simulink model "practice_final_part_5"  (Simulink 8.3)
settings: Solver=ode45  StartTime=0.0  StopTime=20  RelTol=1e-3
undefined symbols (not defined in the file or in its folder): ctrl_est, drawRodMass, P
settings Model: Creator=beard  LastModifiedBy=jhl48
settings DataIOCC: LimitDataPoints=off
settings OptimizationCC: ExpressionDepthLimit=2147483647
settings DebuggingCC: SolverPrmCheckMsg=none  FcnCallInpInsideContextMsg=UseLocalSettings

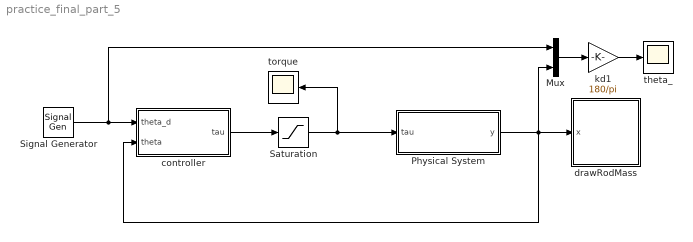
== system practice_final_part_5 ==
  Mux : Mux  Inputs=2
  Physical System : Subsystem
  Saturation : Saturate  UpperLimit=P.tau_max  LowerLimit=-P.tau_max
  Signal Generator : SignalGenerator  WaveForm=square  Amplitude=10*pi/180  Frequency=.1
  controller : Subsystem
  drawRodMass : Subsystem
      mask init:
      | % drawing parameters
      | L = 1;
      | w = 0.01;
      | R = 0.1;
      | H = 1;
      mask Display: image(imread('tv.jpg'))
  kd1 : Gain  Gain=180/pi
  theta_ : Scope
      settings: YMin=-35  YMax=30
  torque : Scope
      settings: YMin=-0.65  YMax=0.2  SaveName=ScopeData2
  wires:
  Mux/1 -> kd1/1
  kd1/1 -> theta_/1
  controller/1(tau) -> Saturation/1
  Signal Generator/1 -> controller/1(theta_d), Mux/1
  Physical System/1(y) -> drawRodMass/1(x), Mux/2, controller/2(theta)
  Saturation/1 -> torque/1, Physical System/1(tau)

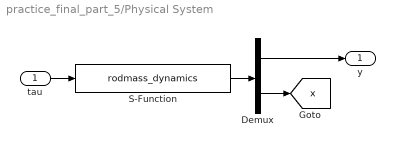
== system practice_final_part_5/Physical System ==
  tau : Inport
  Demux : Demux  Outputs=[1;2]
  S-Function : S-Function  FunctionName=rodmass_dynamics  Parameters=P  EnableBusSupport=off
  y : Outport
  tag scope: x=global
  wires:
  tau/1 -> S-Function/1
  S-Function/1 -> Demux/1
  Demux/2 -> [x]
  Demux/1 -> y/1

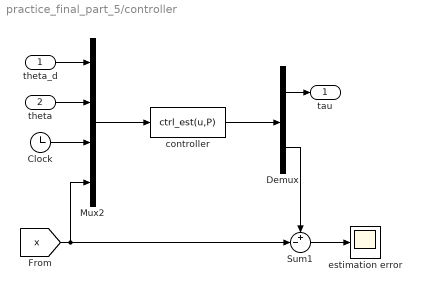
== system practice_final_part_5/controller ==
  theta_d : Inport
  theta : Inport  Port=2
  Clock : Clock
  Demux : Demux  Outputs=[1;2]
  Mux2 : Mux
  Sum1 : Sum  Inputs=+-|
  controller : MATLABFcn  MATLABFcn=ctrl_est(u,P)  OutputDimensions=3  SampleTime=P.Ts
  estimation error : Scope
      settings: YMin=-0.25  YMax=2.5
  tau : Outport
  wires:
  Mux2/1 -> controller/1
  theta_d/1 -> Mux2/1
  theta/1 -> Mux2/2
  Clock/1 -> Mux2/3
  controller/1 -> Demux/1
  Demux/1 -> tau/1
  Demux/2 -> Sum1/1
  Sum1/1 -> estimation error/1
  [x] -> Mux2/4, Sum1/2

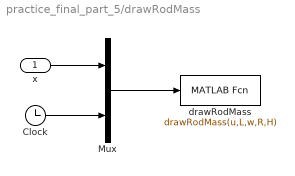
== system practice_final_part_5/drawRodMass ==
  x : Inport
  Clock : Clock
  Mux : Mux  Inputs=2
  drawRodMass : MATLABFcn  MATLABFcn=drawRodMass(u,L,w,R,H)  OutputDimensions=0  SampleTime=0.1
  wires:
  Clock/1 -> Mux/2
  x/1 -> Mux/1
  Mux/1 -> drawRodMass/1
